simulink model "six_plus_six_AcmsteeringV09_main_2lflm"  (R2014a)
settings: Solver=FixedStepDiscrete  StartTime=0.0  StopTime=10.0  FixedStep=0.0005  RelTol=1e-3
InitFcn:
  | Veh_Par_wxt
undefined symbols (not defined in the file or in its folder): acc_spdctl, ag_thr, B, bra_em, bra_pre_gz2, bra_pre_gz34, bra_pre_yd, brakepre_dem_data, brakeTrq_dem_data, bratrq_max, ecucoder_acal, eff_tran, ESP_switch, G, guzhang_lf, guzhang_lm, guzhang_lr, guzhang_rf, guzhang_rm, guzhang_rr, kd1, kd2, ki1, ki2, kp1, kp2, L, myFIS, premax, Radius, RC_switch, s_opt_yi, s_opt_zhuan, s_opt_zhuan_add, s_opt_zhuan_table, spd_map_mot, spd_spdctl, speed_thr_park, TCS_switch, tras_ratio, trq_map_mot, trqmax_yd, trqmax_zx, trqmaxneg, v_gain, v_table, v_thr_park, zhidong_bianmazhi, zhidong_down, zhidong_up, zhidong_youmen, zhuanxiang_bianmazhi, zhuanxiang_down, zhuanxiang_up, zhuanxiang_youmen
libraries: simulink x980, ec5744lib x59, fuzblock x2
(part 15 of 25)

== matlab function six_plus_six_AcmsteeringV09_main_2lflm/MainControl/mode_control/backward/backward/Drive/驱动防滑控制TCS/直行TCS/直行/MATLAB Function ==
  data: s_act_lf input; flag_lf output; s_opt_zhuan input; s_opt_zhuan_add input; flag_lf_pre input int8
function flag_lf = fcn(s_act_lf,s_opt_zhuan,s_opt_zhuan_add,flag_lf_pre)
%#codegen
if s_act_lf>s_opt_zhuan+s_opt_zhuan_add
    flag_lf=int8(1);
elseif s_act_lf<s_opt_zhuan
    flag_lf =int8(0);
else
    flag_lf=int8(flag_lf_pre);
end
end

== matlab function six_plus_six_AcmsteeringV09_main_2lflm/MainControl/mode_control/backward/backward/Drive/驱动防滑控制TCS/直行TCS/直行/MATLAB Function6 ==
  data: s_act_rm input; flag_rm output; s_opt_zhuan input; s_opt_zhuan_add input; flag_rm_pre input int8
function flag_rm = fcn(s_act_rm,s_opt_zhuan,s_opt_zhuan_add,flag_rm_pre)
%#codegen
if s_act_rm>s_opt_zhuan+s_opt_zhuan_add
    flag_rm=int8(1);
elseif s_act_rm<s_opt_zhuan
    flag_rm =int8(0);
else
    flag_rm=int8(flag_rm_pre);
end
end

== matlab function six_plus_six_AcmsteeringV09_main_2lflm/Data_input/5/Enabled
Subsystem/MATLAB Function ==
  data: data1 input; y output; data2 input; data3 input; data4 input
function y = fcn(data1,data2,data3,data4)
%#codegen
y1=data4*256^3+data3*256^2+data2*256+data1;
y=typecast(uint32(y1),'single');
end
% y = u;

== matlab function six_plus_six_AcmsteeringV09_main_2lflm/Data_input/8/Enabled
Subsystem/MATLAB Function1 ==
  data: data1 input; y output; data2 input; data3 input; data4 input
function y = fcn(data1,data2,data3,data4)
%#codegen
y1=data4*256^3+data3*256^2+data2*256+data1;
y=typecast(uint32(y1),'single');
end
% y = u;

== matlab function six_plus_six_AcmsteeringV09_main_2lflm/MainControl/mode_control/backward/backward/Drive/MATLAB Function ==
  data: acc_y input; y output; ag_thr input
function y = fcn(acc_y,ag_thr)
%#codegen
if abs(acc_y)>=ag_thr
    y=int8(0);
else 
    y=int8(1);
end
end

== matlab function six_plus_six_AcmsteeringV09_main_2lflm/MainControl/mode_control/forward/forward/Drive/驱动防滑控制TCS/直行TCS/直行/MATLAB Function5 ==
  data: TCS_switch input; flag_lf1 output; flag_lm1 output; flag_lf input; flag_lm input; flag_lr input; flag_lr1 output; flag_rf input; flag_rm input; flag_rr input; flag_rf1 output; flag_rm1 output; flag_rr1 output
 function [flag_lf1,flag_lm1,flag_lr1,flag_rf1,flag_rm1,flag_rr1] = fcn(TCS_switch,flag_lf,flag_lm,flag_lr,flag_rf,flag_rm,flag_rr)
%#codegen
if TCS_switch==0
    flag_lf1=single(0);
    flag_lm1=single(0);
    flag_lr1=single(0);
    flag_rf1=single(0);
    flag_rm1=single(0);
    flag_rr1=single(0);
else
    flag_lf1=single(flag_lf);
    flag_lm1=single(flag_lm);
    flag_lr1=single(flag_lr);
    flag_rf1=single(flag_rf);
    flag_rm1=single(flag_rm);
    flag_rr1=single(flag_rr);
end
end

== system six_plus_six_AcmsteeringV09_main_2lflm/Data_input/RemoteControl1/Yaokong2 ==
  input : Inport
  Enable : EnablePort
  Demux : Demux  Outputs=8
  LIFEspan_Ad : Sum
  LIFEspan_Convert : DataTypeConversion  OutDataTypeStr=uint32
  LIFEspan_F : Gain
  LIFEspan_L : simulink/Logic and Bit Operations/Bitwise Operator  logicop=AND  UseBitMask=on  BitMask=255  BitMaskRealWorld=Stored Integer
  LIFEspan_O : Constant  Value=0  OutDataTypeStr=single
  LIFEspan_S : ArithShift
  LIFEspan_Sub : Subsystem
  LIFEspan_sat : Saturate  UpperLimit=255  LowerLimit=0
  LIFEspancv : DataTypeConversion
  SA_Ad : Sum
  SA_Convert : DataTypeConversion  OutDataTypeStr=uint32
  SA_F : Gain
  SA_L : simulink/Logic and Bit Operations/Bitwise Operator  logicop=AND  UseBitMask=on  BitMask=255  BitMaskRealWorld=Stored Integer
  SA_O : Constant  Value=0  OutDataTypeStr=single
  SA_S : ArithShift
  SA_Sub : Subsystem
  SA_sat : Saturate  UpperLimit=255  LowerLimit=0
  SAcv : DataTypeConversion
  SD_Ad : Sum
  SD_Convert : DataTypeConversion  OutDataTypeStr=uint32
  SD_F : Gain
  SD_L : simulink/Logic and Bit Operations/Bitwise Operator  logicop=AND  UseBitMask=on  BitMask=255  BitMaskRealWorld=Stored Integer
  SD_O : Constant  Value=0  OutDataTypeStr=single
  SD_S : ArithShift
  SD_Sub : Subsystem
  SD_sat : Saturate  UpperLimit=255  LowerLimit=0
  SDcv : DataTypeConversion
  SE_Ad : Sum
  SE_Convert : DataTypeConversion  OutDataTypeStr=uint32
  SE_F : Gain
  SE_L : simulink/Logic and Bit Operations/Bitwise Operator  logicop=AND  UseBitMask=on  BitMask=255  BitMaskRealWorld=Stored Integer
  SE_O : Constant  Value=0  OutDataTypeStr=single
  SE_S : ArithShift
  SE_Sub : Subsystem
  SE_sat : Saturate  UpperLimit=255  LowerLimit=0
  SEcv : DataTypeConversion
  SH_Ad : Sum
  SH_Convert : DataTypeConversion  OutDataTypeStr=uint32
  SH_F : Gain
  SH_L : simulink/Logic and Bit Operations/Bitwise Operator  logicop=AND  UseBitMask=on  BitMask=255  BitMaskRealWorld=Stored Integer
  SH_O : Constant  Value=0  OutDataTypeStr=single
  SH_S : ArithShift
  SH_Sub : Subsystem
  SH_sat : Saturate  UpperLimit=255  LowerLimit=0
  SHcv : DataTypeConversion
  SH_Out : Outport
  SE_Out : Outport  Port=2
  SD_Out : Outport  Port=3
  SA_Out : Outport  Port=4
  LIFEspan_Out : Outport  Port=5
  wires:
  SH_F/1 -> SH_Ad/1
  SH_O/1 -> SH_Ad/2
  SH_Ad/1 -> SH_sat/1
  SH_sat/1 -> SH_Out/1
  Demux/1 -> SH_Sub/1(In1)
  SH_Sub/1(Out1) -> SH_Convert/1
  SH_Convert/1 -> SH_L/1
  SH_L/1 -> SH_S/1
  SH_S/1 -> SHcv/1
  SHcv/1 -> SH_F/1
  SE_F/1 -> SE_Ad/1
  SE_O/1 -> SE_Ad/2
  SE_Ad/1 -> SE_sat/1
  SE_sat/1 -> SE_Out/1
  Demux/2 -> SE_Sub/1(In1)
  SE_Sub/1(Out1) -> SE_Convert/1
  SE_Convert/1 -> SE_L/1
  SE_L/1 -> SE_S/1
  SE_S/1 -> SEcv/1
  SEcv/1 -> SE_F/1
  SD_F/1 -> SD_Ad/1
  SD_O/1 -> SD_Ad/2
  SD_Ad/1 -> SD_sat/1
  SD_sat/1 -> SD_Out/1
  Demux/3 -> SD_Sub/1(In1)
  SD_Sub/1(Out1) -> SD_Convert/1
  SD_Convert/1 -> SD_L/1
  SD_L/1 -> SD_S/1
  SD_S/1 -> SDcv/1
  SDcv/1 -> SD_F/1
  SA_F/1 -> SA_Ad/1
  SA_O/1 -> SA_Ad/2
  SA_Ad/1 -> SA_sat/1
  SA_sat/1 -> SA_Out/1
  Demux/4 -> SA_Sub/1(In1)
  SA_Sub/1(Out1) -> SA_Convert/1
  SA_Convert/1 -> SA_L/1
  SA_L/1 -> SA_S/1
  SA_S/1 -> SAcv/1
  SAcv/1 -> SA_F/1
  LIFEspan_F/1 -> LIFEspan_Ad/1
  LIFEspan_O/1 -> LIFEspan_Ad/2
  LIFEspan_Ad/1 -> LIFEspan_sat/1
  LIFEspan_sat/1 -> LIFEspan_Out/1
  Demux/5 -> LIFEspan_Sub/1(In1)
  LIFEspan_Sub/1(Out1) -> LIFEspan_Convert/1
  LIFEspan_Convert/1 -> LIFEspan_L/1
  LIFEspan_L/1 -> LIFEspan_S/1
  LIFEspan_S/1 -> LIFEspancv/1
  LIFEspancv/1 -> LIFEspan_F/1
  input/1 -> Demux/1

== system six_plus_six_AcmsteeringV09_main_2lflm/Data_input/RemoteControl2/Yaokong1 ==
  input : Inport
  Enable : EnablePort
  Data Type Conversion : DataTypeConversion
  Data Type Conversion1 : DataTypeConversion
  Demux : Demux  Outputs=8
  Leftstick_leftright_Ad : Sum
  Leftstick_leftright_Convert : DataTypeConversion  OutDataTypeStr=uint32
  Leftstick_leftright_F : Gain
  Leftstick_leftright_L : simulink/Logic and Bit Operations/Bitwise Operator  logicop=AND  UseBitMask=on  BitMask=65535  BitMaskRealWorld=Stored Integer
  Leftstick_leftright_O : Constant  Value=0  OutDataTypeStr=single
  Leftstick_leftright_S : ArithShift
  Leftstick_leftright_Sub : Subsystem
  Leftstick_leftright_sat : Saturate  UpperLimit=65535  LowerLimit=0
  Leftstick_leftrightcv : DataTypeConversion
  Leftstick_leftrightinput1_Ad : Sum
  Leftstick_leftrightinput1_C : Constant  Value=256
  Leftstick_leftrightinput1_P : Product
  Leftstick_updown_Ad : Sum
  Leftstick_updown_Convert : DataTypeConversion  OutDataTypeStr=uint32
  Leftstick_updown_F : Gain
  Leftstick_updown_L : simulink/Logic and Bit Operations/Bitwise Operator  logicop=AND  UseBitMask=on  BitMask=65535  BitMaskRealWorld=Stored Integer
  Leftstick_updown_O : Constant  Value=0  OutDataTypeStr=single
  Leftstick_updown_S : ArithShift
  Leftstick_updown_Sub : Subsystem
  Leftstick_updown_sat : Saturate  UpperLimit=65535  LowerLimit=0
  Leftstick_updowncv : DataTypeConversion
  Leftstick_updowninput3_Ad : Sum
  Leftstick_updowninput3_C : Constant  Value=256
  Leftstick_updowninput3_P : Product
  Rightstick_leftright_Ad : Sum
  Rightstick_leftright_Convert : DataTypeConversion  OutDataTypeStr=uint32
  Rightstick_leftright_F : Gain
  Rightstick_leftright_L : simulink/Logic and Bit Operations/Bitwise Operator  logicop=AND  UseBitMask=on  BitMask=65535  BitMaskRealWorld=Stored Integer
  Rightstick_leftright_O : Constant  Value=0  OutDataTypeStr=single
  Rightstick_leftright_S : ArithShift
  Rightstick_leftright_Sub : Subsystem
  Rightstick_leftright_sat : Saturate  UpperLimit=65535  LowerLimit=0
  Rightstick_leftrightcv : DataTypeConversion
  Rightstick_leftrightinput5_Ad : Sum
  Rightstick_leftrightinput5_C : Constant  Value=256
  Rightstick_leftrightinput5_P : Product
  Rightstick_updown_Ad : Sum
  Rightstick_updown_Convert : DataTypeConversion  OutDataTypeStr=uint32
  Rightstick_updown_F : Gain
  Rightstick_updown_L : simulink/Logic and Bit Operations/Bitwise Operator  logicop=AND  UseBitMask=on  BitMask=65535  BitMaskRealWorld=Stored Integer
  Rightstick_updown_O : Constant  Value=0  OutDataTypeStr=single
  Rightstick_updown_S : ArithShift
  Rightstick_updown_Sub : Subsystem
  Rightstick_updown_sat : Saturate  UpperLimit=65535  LowerLimit=0
  Rightstick_updowncv : DataTypeConversion
  Rightstick_updowninput7_Ad : Sum
  Rightstick_updowninput7_C : Constant  Value=256
  Rightstick_updowninput7_P : Product
  Rightstick_updown_Out : Outport
  Rightstick_leftright_Out : Outport  Port=2
  Leftstick_updown_Out : Outport  Port=3
  Leftstick_leftright_Out : Outport  Port=4
  wires:
  Rightstick_updown_F/1 -> Rightstick_updown_Ad/1
  Rightstick_updown_O/1 -> Rightstick_updown_Ad/2
  Rightstick_updown_Ad/1 -> Rightstick_updown_sat/1
  Rightstick_updown_sat/1 -> Rightstick_updown_Out/1
  Demux/7 -> Rightstick_updowninput7_P/1
  Rightstick_updowninput7_C/1 -> Rightstick_updowninput7_P/2
  Rightstick_updowninput7_P/1 -> Rightstick_updowninput7_Ad/1
  Demux/8 -> Rightstick_updowninput7_Ad/2
  Rightstick_updowninput7_Ad/1 -> Rightstick_updown_Sub/1(In1)
  Rightstick_updown_Sub/1(Out1) -> Rightstick_updown_Convert/1
  Rightstick_updown_Convert/1 -> Rightstick_updown_L/1
  Rightstick_updown_L/1 -> Rightstick_updown_S/1
  Rightstick_updown_S/1 -> Rightstick_updowncv/1
  Rightstick_updowncv/1 -> Rightstick_updown_F/1
  Rightstick_leftright_F/1 -> Rightstick_leftright_Ad/1
  Rightstick_leftright_O/1 -> Rightstick_leftright_Ad/2
  Rightstick_leftright_Ad/1 -> Rightstick_leftright_sat/1
  Rightstick_leftright_sat/1 -> Rightstick_leftright_Out/1
  Demux/5 -> Rightstick_leftrightinput5_P/1
  Rightstick_leftrightinput5_C/1 -> Rightstick_leftrightinput5_P/2
  Rightstick_leftrightinput5_P/1 -> Rightstick_leftrightinput5_Ad/1
  Demux/6 -> Rightstick_leftrightinput5_Ad/2
  Rightstick_leftrightinput5_Ad/1 -> Rightstick_leftright_Sub/1(In1)
  Rightstick_leftright_Sub/1(Out1) -> Rightstick_leftright_Convert/1
  Rightstick_leftright_Convert/1 -> Rightstick_leftright_L/1
  Rightstick_leftright_L/1 -> Rightstick_leftright_S/1
  Rightstick_leftright_S/1 -> Rightstick_leftrightcv/1
  Rightstick_leftrightcv/1 -> Rightstick_leftright_F/1
  Leftstick_updown_F/1 -> Leftstick_updown_Ad/1
  Leftstick_updown_O/1 -> Leftstick_updown_Ad/2
  Leftstick_updown_Ad/1 -> Leftstick_updown_sat/1
  Leftstick_updown_sat/1 -> Leftstick_updown_Out/1
  Demux/3 -> Data Type Conversion/1
  Leftstick_updowninput3_C/1 -> Leftstick_updowninput3_P/2
  Leftstick_updowninput3_P/1 -> Leftstick_updowninput3_Ad/1
  Demux/4 -> Data Type Conversion1/1
  Leftstick_updowninput3_Ad/1 -> Leftstick_updown_Sub/1(In1)
  Leftstick_updown_Sub/1(Out1) -> Leftstick_updown_Convert/1
  Leftstick_updown_Convert/1 -> Leftstick_updown_L/1
  Leftstick_updown_L/1 -> Leftstick_updown_S/1
  Leftstick_updown_S/1 -> Leftstick_updowncv/1
  Leftstick_updowncv/1 -> Leftstick_updown_F/1
  Leftstick_leftright_F/1 -> Leftstick_leftright_Ad/1
  Leftstick_leftright_O/1 -> Leftstick_leftright_Ad/2
  Leftstick_leftright_Ad/1 -> Leftstick_leftright_sat/1
  Leftstick_leftright_sat/1 -> Leftstick_leftright_Out/1
  Demux/1 -> Leftstick_leftrightinput1_P/1
  Leftstick_leftrightinput1_C/1 -> Leftstick_leftrightinput1_P/2
  Leftstick_leftrightinput1_P/1 -> Leftstick_leftrightinput1_Ad/1
  Demux/2 -> Leftstick_leftrightinput1_Ad/2
  Leftstick_leftrightinput1_Ad/1 -> Leftstick_leftright_Sub/1(In1)
  Leftstick_leftright_Sub/1(Out1) -> Leftstick_leftright_Convert/1
  Leftstick_leftright_Convert/1 -> Leftstick_leftright_L/1
  Leftstick_leftright_L/1 -> Leftstick_leftright_S/1
  Leftstick_leftright_S/1 -> Leftstick_leftrightcv/1
  Leftstick_leftrightcv/1 -> Leftstick_leftright_F/1
  input/1 -> Demux/1
  Data Type Conversion/1 -> Leftstick_updowninput3_P/1
  Data Type Conversion1/1 -> Leftstick_updowninput3_Ad/2

== system six_plus_six_AcmsteeringV09_main_2lflm/MainControl/mode_control/Park ==
  Signals : Inport
  Action Port : ActionPort  ActionType=case
  Mux : Mux  Inputs=10
  park : Subsystem
  park_dem : Outport
  wires:
  Signals/1 -> park/1(Signals)
  Mux/1 -> park_dem/1
  park/9(motec_position_3) -> Mux/9
  park/10(motec_position_4) -> Mux/10
  park/1(mot_lf) -> Mux/1
  park/2(mot_lm) -> Mux/2
  park/5(mot_rm) -> Mux/5
  park/4(mot_rf) -> Mux/4
  park/3(mot_lr) -> Mux/3
  park/7(motec_position_1) -> Mux/7
  park/8(motec_position_2) -> Mux/8
  park/6(mot_rr) -> Mux/6

== system six_plus_six_AcmsteeringV09_main_2lflm/MainControl/mode_control/backward ==
  Signals : Inport
  Action Port : ActionPort  ActionType=case
  backward : Subsystem
  backward_dem : Outport
  wires:
  Signals/1 -> backward/1(Signals)
  backward/1(backward_dem) -> backward_dem/1

== system six_plus_six_AcmsteeringV09_main_2lflm/MainControl/mode_control/center_steer ==
  Signals : Inport
  Action Port : ActionPort  ActionType=case
  Mux : Mux  Inputs=10
  center_steer : Subsystem
  center_steer_dem : Outport
  wires:
  Mux/1 -> center_steer_dem/1
  Signals/1 -> center_steer/1(Signals)
  center_steer/6(mot_rr) -> Mux/6
  center_steer/1(mot_lf) -> Mux/1
  center_steer/4(mot_rf) -> Mux/4
  center_steer/3(mot_lr) -> Mux/3
  center_steer/5(mot_rm) -> Mux/5
  center_steer/2(mot_lm) -> Mux/2
  center_steer/7(motec_position_1) -> Mux/7
  center_steer/8(motec_position_2) -> Mux/8
  center_steer/10(motec_position_4) -> Mux/10
  center_steer/9(motec_position_3) -> Mux/9

== system six_plus_six_AcmsteeringV09_main_2lflm/MainControl/mode_control/emergency_stop ==
  Signals : Inport
  Action Port : ActionPort  ActionType=case
  Mux : Mux  Inputs=10
  emergency_stop : Subsystem
  emergency_stop_dem : Outport
  wires:
  Mux/1 -> emergency_stop_dem/1
  Signals/1 -> emergency_stop/1(Signals)
  emergency_stop/8(motec_position_2) -> Mux/8
  emergency_stop/9(motec_position_3) -> Mux/9
  emergency_stop/10(motec_position_4) -> Mux/10
  emergency_stop/7(motec_position_1) -> Mux/7
  emergency_stop/3(mot_lr) -> Mux/3
  emergency_stop/1(mot_lf) -> Mux/1
  emergency_stop/2(mot_lm) -> Mux/2
  emergency_stop/5(mot_rm) -> Mux/5
  emergency_stop/6(mot_rr) -> Mux/6
  emergency_stop/4(mot_rf) -> Mux/4

== system six_plus_six_AcmsteeringV09_main_2lflm/MainControl/mode_control/forward ==
  Signals : Inport
  Action Port : ActionPort  ActionType=case
  forward : Subsystem
  forward_dem : Outport
  wires:
  Signals/1 -> forward/1(Signals)
  forward/1(forward_dem) -> forward_dem/1

== system six_plus_six_AcmsteeringV09_main_2lflm/MainControl/mode_control/neutral ==
  Signals : Inport
  Action Port : ActionPort  ActionType=case
  Mux : Mux  Inputs=10
  neutral : Subsystem
  neutral_dem : Outport
  wires:
  Mux/1 -> neutral_dem/1
  Signals/1 -> neutral/1(Signals)
  neutral/3(mot_lr) -> Mux/3
  neutral/5(mot_rm) -> Mux/5
  neutral/6(mot_rr) -> Mux/6
  neutral/2(mot_lm) -> Mux/2
  neutral/1(mot_lf) -> Mux/1
  neutral/4(mot_rf) -> Mux/4
  neutral/7(motec_position_1) -> Mux/7
  neutral/8(motec_position_2) -> Mux/8
  neutral/10(motec_position_4) -> Mux/10
  neutral/9(motec_position_3) -> Mux/9

== system six_plus_six_AcmsteeringV09_main_2lflm/Subsystem/VCU1/VCU1_CtrlModel ==
  VCU1_CtrlModel : Inport
  Constant{2..8} (7 alike) : Constant  Value=0  OutDataTypeStr=uint8
  VCU1_CtrlModelRon : Rounding  Operator=round
  VCU1_CtrlModel_1sat : Saturate  UpperLimit=4  LowerLimit=0
  VCU1_CtrlModel_Convert : DataTypeConversion  OutDataTypeStr=uint8
  VCU1_CtrlModel_Convert1 : DataTypeConversion  OutDataTypeStr=uint32
  VCU1_CtrlModel_D : Product  Inputs=*/
  VCU1_CtrlModel_F : Constant  OutDataTypeStr=single
  VCU1_CtrlModel_L : simulink/Logic and Bit Operations/Bitwise Operator  logicop=AND  UseBitMask=on  BitMask=4  BitMaskRealWorld=Stored Integer
  VCU1_CtrlModel_O : Constant  Value=0  OutDataTypeStr=single
  VCU1_CtrlModel_S : ArithShift  BitShiftNumber=-2
  VCU1_CtrlModel_sat : Saturate  UpperLimit=1  LowerLimit=0
  VCU1_CtrlModel_st : Sum  Inputs=+-
  output1 : Outport
  output2 : Outport  Port=2
  output3 : Outport  Port=3
  output4 : Outport  Port=4
  output5 : Outport  Port=5
  output6 : Outport  Port=6
  output7 : Outport  Port=7
  output8 : Outport  Port=8
  wires:
  VCU1_CtrlModel/1 -> VCU1_CtrlModel_sat/1
  VCU1_CtrlModel_sat/1 -> VCU1_CtrlModel_st/1
  VCU1_CtrlModel_O/1 -> VCU1_CtrlModel_st/2
  VCU1_CtrlModel_st/1 -> VCU1_CtrlModel_D/1
  VCU1_CtrlModel_F/1 -> VCU1_CtrlModel_D/2
  VCU1_CtrlModel_D/1 -> VCU1_CtrlModelRon/1
  VCU1_CtrlModelRon/1 -> VCU1_CtrlModel_S/1
  VCU1_CtrlModel_S/1 -> VCU1_CtrlModel_1sat/1
  VCU1_CtrlModel_1sat/1 -> VCU1_CtrlModel_Convert1/1
  VCU1_CtrlModel_Convert1/1 -> VCU1_CtrlModel_L/1
  VCU1_CtrlModel_L/1 -> VCU1_CtrlModel_Convert/1
  VCU1_CtrlModel_Convert/1 -> output1/1
  Constant2/1 -> output2/1
  Constant3/1 -> output3/1
  Constant4/1 -> output4/1
  Constant5/1 -> output5/1
  Constant6/1 -> output6/1
  Constant7/1 -> output7/1
  Constant8/1 -> output8/1

== system six_plus_six_AcmsteeringV09_main_2lflm/Subsystem/VCU1/VCU1_EnableReq ==
  VCU1_EnableReq : Inport
  Constant{2..8} (7 alike) : Constant  Value=0  OutDataTypeStr=uint8
  VCU1_EnableReqRon : Rounding  Operator=round
  VCU1_EnableReq_1sat : Saturate  UpperLimit=3  LowerLimit=0
  VCU1_EnableReq_Convert : DataTypeConversion  OutDataTypeStr=uint8
  VCU1_EnableReq_Convert1 : DataTypeConversion  OutDataTypeStr=uint32
  VCU1_EnableReq_D : Product  Inputs=*/
  VCU1_EnableReq_F : Constant  OutDataTypeStr=single
  VCU1_EnableReq_L : simulink/Logic and Bit Operations/Bitwise Operator  logicop=AND  UseBitMask=on  BitMask=3  BitMaskRealWorld=Stored Integer
  VCU1_EnableReq_O : Constant  Value=0  OutDataTypeStr=single
  VCU1_EnableReq_S : ArithShift
  VCU1_EnableReq_sat : Saturate  UpperLimit=3  LowerLimit=0
  VCU1_EnableReq_st : Sum  Inputs=+-
  output1 : Outport
  output2 : Outport  Port=2
  output3 : Outport  Port=3
  output4 : Outport  Port=4
  output5 : Outport  Port=5
  output6 : Outport  Port=6
  output7 : Outport  Port=7
  output8 : Outport  Port=8
  wires:
  VCU1_EnableReq/1 -> VCU1_EnableReq_sat/1
  VCU1_EnableReq_sat/1 -> VCU1_EnableReq_st/1
  VCU1_EnableReq_O/1 -> VCU1_EnableReq_st/2
  VCU1_EnableReq_st/1 -> VCU1_EnableReq_D/1
  VCU1_EnableReq_F/1 -> VCU1_EnableReq_D/2
  VCU1_EnableReq_D/1 -> VCU1_EnableReqRon/1
  VCU1_EnableReqRon/1 -> VCU1_EnableReq_S/1
  VCU1_EnableReq_S/1 -> VCU1_EnableReq_1sat/1
  VCU1_EnableReq_1sat/1 -> VCU1_EnableReq_Convert1/1
  VCU1_EnableReq_Convert1/1 -> VCU1_EnableReq_L/1
  VCU1_EnableReq_L/1 -> VCU1_EnableReq_Convert/1
  VCU1_EnableReq_Convert/1 -> output1/1
  Constant2/1 -> output2/1
  Constant3/1 -> output3/1
  Constant4/1 -> output4/1
  Constant5/1 -> output5/1
  Constant6/1 -> output6/1
  Constant7/1 -> output7/1
  Constant8/1 -> output8/1

== system six_plus_six_AcmsteeringV09_main_2lflm/Subsystem/VCU1/VCU1_GearCmd ==
  VCU1_GearCmd : Inport
  Constant{2..8} (7 alike) : Constant  Value=0  OutDataTypeStr=uint8
  VCU1_GearCmdRon : Rounding  Operator=round
  VCU1_GearCmd_1sat : Saturate  UpperLimit=24  LowerLimit=0
  VCU1_GearCmd_Convert : DataTypeConversion  OutDataTypeStr=uint8
  VCU1_GearCmd_Convert1 : DataTypeConversion  OutDataTypeStr=uint32
  VCU1_GearCmd_D : Product  Inputs=*/
  VCU1_GearCmd_F : Constant  OutDataTypeStr=single
  VCU1_GearCmd_L : simulink/Logic and Bit Operations/Bitwise Operator  logicop=AND  UseBitMask=on  BitMask=24  BitMaskRealWorld=Stored Integer
  VCU1_GearCmd_O : Constant  Value=0  OutDataTypeStr=single
  VCU1_GearCmd_S : ArithShift  BitShiftNumber=-3
  VCU1_GearCmd_sat : Saturate  UpperLimit=3  LowerLimit=0
  VCU1_GearCmd_st : Sum  Inputs=+-
  output1 : Outport
  output2 : Outport  Port=2
  output3 : Outport  Port=3
  output4 : Outport  Port=4
  output5 : Outport  Port=5
  output6 : Outport  Port=6
  output7 : Outport  Port=7
  output8 : Outport  Port=8
  wires:
  VCU1_GearCmd/1 -> VCU1_GearCmd_sat/1
  VCU1_GearCmd_sat/1 -> VCU1_GearCmd_st/1
  VCU1_GearCmd_O/1 -> VCU1_GearCmd_st/2
  VCU1_GearCmd_st/1 -> VCU1_GearCmd_D/1
  VCU1_GearCmd_F/1 -> VCU1_GearCmd_D/2
  VCU1_GearCmd_D/1 -> VCU1_GearCmdRon/1
  VCU1_GearCmdRon/1 -> VCU1_GearCmd_S/1
  VCU1_GearCmd_S/1 -> VCU1_GearCmd_1sat/1
  VCU1_GearCmd_1sat/1 -> VCU1_GearCmd_Convert1/1
  VCU1_GearCmd_Convert1/1 -> VCU1_GearCmd_L/1
  VCU1_GearCmd_L/1 -> VCU1_GearCmd_Convert/1
  VCU1_GearCmd_Convert/1 -> output1/1
  Constant2/1 -> output2/1
  Constant3/1 -> output3/1
  Constant4/1 -> output4/1
  Constant5/1 -> output5/1
  Constant6/1 -> output6/1
  Constant7/1 -> output7/1
  Constant8/1 -> output8/1

== system six_plus_six_AcmsteeringV09_main_2lflm/Subsystem/VCU1/VCU1_LifeCnt ==
  VCU1_LifeCnt : Inport
  Constant{1..7} (7 alike) : Constant  Value=0  OutDataTypeStr=uint8
  VCU1_LifeCntRon : Rounding  Operator=round
  VCU1_LifeCnt_1sat : Saturate  UpperLimit=255  LowerLimit=0
  VCU1_LifeCnt_Convert : DataTypeConversion  OutDataTypeStr=uint8
  VCU1_LifeCnt_Convert1 : DataTypeConversion  OutDataTypeStr=uint32
  VCU1_LifeCnt_D : Product  Inputs=*/
  VCU1_LifeCnt_F : Constant  OutDataTypeStr=single
  VCU1_LifeCnt_L : simulink/Logic and Bit Operations/Bitwise Operator  logicop=AND  UseBitMask=on  BitMask=255  BitMaskRealWorld=Stored Integer
  VCU1_LifeCnt_O : Constant  Value=0  OutDataTypeStr=single
  VCU1_LifeCnt_S : ArithShift
  VCU1_LifeCnt_sat : Saturate  UpperLimit=255  LowerLimit=0
  VCU1_LifeCnt_st : Sum  Inputs=+-
  output1 : Outport
  output2 : Outport  Port=2
  output3 : Outport  Port=3
  output4 : Outport  Port=4
  output5 : Outport  Port=5
  output6 : Outport  Port=6
  output7 : Outport  Port=7
  output8 : Outport  Port=8
  wires:
  VCU1_LifeCnt/1 -> VCU1_LifeCnt_sat/1
  VCU1_LifeCnt_sat/1 -> VCU1_LifeCnt_st/1
  VCU1_LifeCnt_O/1 -> VCU1_LifeCnt_st/2
  VCU1_LifeCnt_st/1 -> VCU1_LifeCnt_D/1
  VCU1_LifeCnt_F/1 -> VCU1_LifeCnt_D/2
  VCU1_LifeCnt_D/1 -> VCU1_LifeCntRon/1
  VCU1_LifeCntRon/1 -> VCU1_LifeCnt_S/1
  VCU1_LifeCnt_S/1 -> VCU1_LifeCnt_1sat/1
  VCU1_LifeCnt_1sat/1 -> VCU1_LifeCnt_Convert1/1
  VCU1_LifeCnt_Convert1/1 -> VCU1_LifeCnt_L/1
  VCU1_LifeCnt_L/1 -> VCU1_LifeCnt_Convert/1
  VCU1_LifeCnt_Convert/1 -> output8/1
  Constant1/1 -> output1/1
  Constant2/1 -> output2/1
  Constant3/1 -> output3/1
  Constant4/1 -> output4/1
  Constant5/1 -> output5/1
  Constant6/1 -> output6/1
  Constant7/1 -> output7/1

== system six_plus_six_AcmsteeringV09_main_2lflm/Subsystem/VCU1/VCU1_SpeedMax ==
  VCU1_SpeedMax : Inport
  Constant{1,4..8} (6 alike) : Constant  Value=0  OutDataTypeStr=uint8
  VCU1_SpeedMaxBitCov : DataTypeConversion  OutDataTypeStr=uint8
  VCU1_SpeedMaxCOV : DataTypeConversion  OutDataTypeStr=uint8
  VCU1_SpeedMaxRon : Rounding  Operator=round
  VCU1_SpeedMax_1sat : Saturate  UpperLimit=65535  LowerLimit=0
  VCU1_SpeedMax_And : simulink/Logic and Bit Operations/Bitwise Operator  logicop=AND  UseBitMask=off  NumInputPorts=2  BitMask=bin2dec('11011001')  BitMaskRealWorld=Stored Integer
  VCU1_SpeedMax_And_C : Constant  Value=255  OutDataTypeStr=uint32
  VCU1_SpeedMax_Convert : DataTypeConversion  OutDataTypeStr=uint32
  VCU1_SpeedMax_D : Product  Inputs=*/
  VCU1_SpeedMax_D1 : Product  Inputs=*/
  VCU1_SpeedMax_F : Constant  OutDataTypeStr=single
  VCU1_SpeedMax_L : simulink/Logic and Bit Operations/Bitwise Operator  logicop=AND  UseBitMask=on  BitMask=65535  BitMaskRealWorld=Stored Integer
  VCU1_SpeedMax_O : Constant  Value=0  OutDataTypeStr=single
  VCU1_SpeedMax_S : ArithShift
  VCU1_SpeedMax_sat : Saturate  UpperLimit=10000  LowerLimit=0
  VCU1_SpeedMax_st : Sum  Inputs=+-
  VCU1_SpeedMaxoutput2_C : Constant  Value=256
  output1 : Outport
  output2 : Outport  Port=2
  output3 : Outport  Port=3
  output4 : Outport  Port=4
  output5 : Outport  Port=5
  output6 : Outport  Port=6
  output7 : Outport  Port=7
  output8 : Outport  Port=8
  wires:
  VCU1_SpeedMax/1 -> VCU1_SpeedMax_sat/1
  VCU1_SpeedMax_sat/1 -> VCU1_SpeedMax_st/1
  VCU1_SpeedMax_O/1 -> VCU1_SpeedMax_st/2
  VCU1_SpeedMax_st/1 -> VCU1_SpeedMax_D/1
  VCU1_SpeedMax_F/1 -> VCU1_SpeedMax_D/2
  VCU1_SpeedMax_D/1 -> VCU1_SpeedMaxRon/1
  VCU1_SpeedMaxRon/1 -> VCU1_SpeedMax_S/1
  VCU1_SpeedMax_S/1 -> VCU1_SpeedMax_1sat/1
  VCU1_SpeedMax_1sat/1 -> VCU1_SpeedMax_Convert/1
  VCU1_SpeedMax_Convert/1 -> VCU1_SpeedMax_L/1
  VCU1_SpeedMax_L/1 -> VCU1_SpeedMax_D1/1, VCU1_SpeedMax_And/1
  VCU1_SpeedMaxoutput2_C/1 -> VCU1_SpeedMax_D1/2
  VCU1_SpeedMax_D1/1 -> VCU1_SpeedMaxCOV/1
  VCU1_SpeedMaxCOV/1 -> output2/1
  VCU1_SpeedMax_And_C/1 -> VCU1_SpeedMax_And/2
  VCU1_SpeedMax_And/1 -> VCU1_SpeedMaxBitCov/1
  VCU1_SpeedMaxBitCov/1 -> output3/1
  Constant1/1 -> output1/1
  Constant4/1 -> output4/1
  Constant5/1 -> output5/1
  Constant6/1 -> output6/1
  Constant7/1 -> output7/1
  Constant8/1 -> output8/1

== system six_plus_six_AcmsteeringV09_main_2lflm/Subsystem/VCU1/VCU1_TorqueRef ==
  VCU1_TorqueRef : Inport
  Constant{1..3,6..8} (6 alike) : Constant  Value=0  OutDataTypeStr=uint8
  VCU1_TorqueRefBitCov : DataTypeConversion  OutDataTypeStr=uint8
  VCU1_TorqueRefCOV : DataTypeConversion  OutDataTypeStr=uint8
  VCU1_TorqueRefRon : Rounding  Operator=round
  VCU1_TorqueRef_1sat : Saturate  UpperLimit=65535  LowerLimit=0
  VCU1_TorqueRef_And : simulink/Logic and Bit Operations/Bitwise Operator  logicop=AND  UseBitMask=off  NumInputPorts=2  BitMask=bin2dec('11011001')  BitMaskRealWorld=Stored Integer
  VCU1_TorqueRef_And_C : Constant  Value=255  OutDataTypeStr=uint32
  VCU1_TorqueRef_Convert : DataTypeConversion  OutDataTypeStr=uint32
  VCU1_TorqueRef_D : Product  Inputs=*/
  VCU1_TorqueRef_D1 : Product  Inputs=*/
  VCU1_TorqueRef_F : Constant  Value=0.1  OutDataTypeStr=single
  VCU1_TorqueRef_L : simulink/Logic and Bit Operations/Bitwise Operator  logicop=AND  UseBitMask=on  BitMask=65535  BitMaskRealWorld=Stored Integer
  VCU1_TorqueRef_O : Constant  Value=-1000  OutDataTypeStr=single
  VCU1_TorqueRef_S : ArithShift
  VCU1_TorqueRef_sat : Saturate  UpperLimit=1000  LowerLimit=-1000
  VCU1_TorqueRef_st : Sum  Inputs=+-
  VCU1_TorqueRefoutput4_C : Constant  Value=256
  output1 : Outport
  output2 : Outport  Port=2
  output3 : Outport  Port=3
  output4 : Outport  Port=4
  output5 : Outport  Port=5
  output6 : Outport  Port=6
  output7 : Outport  Port=7
  output8 : Outport  Port=8
  wires:
  VCU1_TorqueRef/1 -> VCU1_TorqueRef_sat/1
  VCU1_TorqueRef_sat/1 -> VCU1_TorqueRef_st/1
  VCU1_TorqueRef_O/1 -> VCU1_TorqueRef_st/2
  VCU1_TorqueRef_st/1 -> VCU1_TorqueRef_D/1
  VCU1_TorqueRef_F/1 -> VCU1_TorqueRef_D/2
  VCU1_TorqueRef_D/1 -> VCU1_TorqueRefRon/1
  VCU1_TorqueRefRon/1 -> VCU1_TorqueRef_S/1
  VCU1_TorqueRef_S/1 -> VCU1_TorqueRef_1sat/1
  VCU1_TorqueRef_1sat/1 -> VCU1_TorqueRef_Convert/1
  VCU1_TorqueRef_Convert/1 -> VCU1_TorqueRef_L/1
  VCU1_TorqueRef_L/1 -> VCU1_TorqueRef_D1/1, VCU1_TorqueRef_And/1
  VCU1_TorqueRefoutput4_C/1 -> VCU1_TorqueRef_D1/2
  VCU1_TorqueRef_D1/1 -> VCU1_TorqueRefCOV/1
  VCU1_TorqueRefCOV/1 -> output4/1
  VCU1_TorqueRef_And_C/1 -> VCU1_TorqueRef_And/2
  VCU1_TorqueRef_And/1 -> VCU1_TorqueRefBitCov/1
  VCU1_TorqueRefBitCov/1 -> output5/1
  Constant1/1 -> output1/1
  Constant2/1 -> output2/1
  Constant3/1 -> output3/1
  Constant6/1 -> output6/1
  Constant7/1 -> output7/1
  Constant8/1 -> output8/1

== system six_plus_six_AcmsteeringV09_main_2lflm/Subsystem/VCU2/VCU1_CtrlModel ==
  VCU1_CtrlModel : Inport
  Constant{2..8} (7 alike) : Constant  Value=0  OutDataTypeStr=uint8
  VCU1_CtrlModelRon : Rounding  Operator=round
  VCU1_CtrlModel_1sat : Saturate  UpperLimit=4  LowerLimit=0
  VCU1_CtrlModel_Convert : DataTypeConversion  OutDataTypeStr=uint8
  VCU1_CtrlModel_Convert1 : DataTypeConversion  OutDataTypeStr=uint32
  VCU1_CtrlModel_D : Product  Inputs=*/
  VCU1_CtrlModel_F : Constant  OutDataTypeStr=single
  VCU1_CtrlModel_L : simulink/Logic and Bit Operations/Bitwise Operator  logicop=AND  UseBitMask=on  BitMask=4  BitMaskRealWorld=Stored Integer
  VCU1_CtrlModel_O : Constant  Value=0  OutDataTypeStr=single
  VCU1_CtrlModel_S : ArithShift  BitShiftNumber=-2
  VCU1_CtrlModel_sat : Saturate  UpperLimit=1  LowerLimit=0
  VCU1_CtrlModel_st : Sum  Inputs=+-
  output1 : Outport
  output2 : Outport  Port=2
  output3 : Outport  Port=3
  output4 : Outport  Port=4
  output5 : Outport  Port=5
  output6 : Outport  Port=6
  output7 : Outport  Port=7
  output8 : Outport  Port=8
  wires:
  VCU1_CtrlModel/1 -> VCU1_CtrlModel_sat/1
  VCU1_CtrlModel_sat/1 -> VCU1_CtrlModel_st/1
  VCU1_CtrlModel_O/1 -> VCU1_CtrlModel_st/2
  VCU1_CtrlModel_st/1 -> VCU1_CtrlModel_D/1
  VCU1_CtrlModel_F/1 -> VCU1_CtrlModel_D/2
  VCU1_CtrlModel_D/1 -> VCU1_CtrlModelRon/1
  VCU1_CtrlModelRon/1 -> VCU1_CtrlModel_S/1
  VCU1_CtrlModel_S/1 -> VCU1_CtrlModel_1sat/1
  VCU1_CtrlModel_1sat/1 -> VCU1_CtrlModel_Convert1/1
  VCU1_CtrlModel_Convert1/1 -> VCU1_CtrlModel_L/1
  VCU1_CtrlModel_L/1 -> VCU1_CtrlModel_Convert/1
  VCU1_CtrlModel_Convert/1 -> output1/1
  Constant2/1 -> output2/1
  Constant3/1 -> output3/1
  Constant4/1 -> output4/1
  Constant5/1 -> output5/1
  Constant6/1 -> output6/1
  Constant7/1 -> output7/1
  Constant8/1 -> output8/1

== system six_plus_six_AcmsteeringV09_main_2lflm/Subsystem/VCU2/VCU1_EnableReq ==
  VCU1_EnableReq : Inport
  Constant{2..8} (7 alike) : Constant  Value=0  OutDataTypeStr=uint8
  VCU1_EnableReqRon : Rounding  Operator=round
  VCU1_EnableReq_1sat : Saturate  UpperLimit=3  LowerLimit=0
  VCU1_EnableReq_Convert : DataTypeConversion  OutDataTypeStr=uint8
  VCU1_EnableReq_Convert1 : DataTypeConversion  OutDataTypeStr=uint32
  VCU1_EnableReq_D : Product  Inputs=*/
  VCU1_EnableReq_F : Constant  OutDataTypeStr=single
  VCU1_EnableReq_L : simulink/Logic and Bit Operations/Bitwise Operator  logicop=AND  UseBitMask=on  BitMask=3  BitMaskRealWorld=Stored Integer
  VCU1_EnableReq_O : Constant  Value=0  OutDataTypeStr=single
  VCU1_EnableReq_S : ArithShift
  VCU1_EnableReq_sat : Saturate  UpperLimit=3  LowerLimit=0
  VCU1_EnableReq_st : Sum  Inputs=+-
  output1 : Outport
  output2 : Outport  Port=2
  output3 : Outport  Port=3
  output4 : Outport  Port=4
  output5 : Outport  Port=5
  output6 : Outport  Port=6
  output7 : Outport  Port=7
  output8 : Outport  Port=8
  wires:
  VCU1_EnableReq/1 -> VCU1_EnableReq_sat/1
  VCU1_EnableReq_sat/1 -> VCU1_EnableReq_st/1
  VCU1_EnableReq_O/1 -> VCU1_EnableReq_st/2
  VCU1_EnableReq_st/1 -> VCU1_EnableReq_D/1
  VCU1_EnableReq_F/1 -> VCU1_EnableReq_D/2
  VCU1_EnableReq_D/1 -> VCU1_EnableReqRon/1
  VCU1_EnableReqRon/1 -> VCU1_EnableReq_S/1
  VCU1_EnableReq_S/1 -> VCU1_EnableReq_1sat/1
  VCU1_EnableReq_1sat/1 -> VCU1_EnableReq_Convert1/1
  VCU1_EnableReq_Convert1/1 -> VCU1_EnableReq_L/1
  VCU1_EnableReq_L/1 -> VCU1_EnableReq_Convert/1
  VCU1_EnableReq_Convert/1 -> output1/1
  Constant2/1 -> output2/1
  Constant3/1 -> output3/1
  Constant4/1 -> output4/1
  Constant5/1 -> output5/1
  Constant6/1 -> output6/1
  Constant7/1 -> output7/1
  Constant8/1 -> output8/1

== system six_plus_six_AcmsteeringV09_main_2lflm/Subsystem/VCU2/VCU1_GearCmd ==
  VCU1_GearCmd : Inport
  Constant{2..8} (7 alike) : Constant  Value=0  OutDataTypeStr=uint8
  VCU1_GearCmdRon : Rounding  Operator=round
  VCU1_GearCmd_1sat : Saturate  UpperLimit=24  LowerLimit=0
  VCU1_GearCmd_Convert : DataTypeConversion  OutDataTypeStr=uint8
  VCU1_GearCmd_Convert1 : DataTypeConversion  OutDataTypeStr=uint32
  VCU1_GearCmd_D : Product  Inputs=*/
  VCU1_GearCmd_F : Constant  OutDataTypeStr=single
  VCU1_GearCmd_L : simulink/Logic and Bit Operations/Bitwise Operator  logicop=AND  UseBitMask=on  BitMask=24  BitMaskRealWorld=Stored Integer
  VCU1_GearCmd_O : Constant  Value=0  OutDataTypeStr=single
  VCU1_GearCmd_S : ArithShift  BitShiftNumber=-3
  VCU1_GearCmd_sat : Saturate  UpperLimit=3  LowerLimit=0
  VCU1_GearCmd_st : Sum  Inputs=+-
  output1 : Outport
  output2 : Outport  Port=2
  output3 : Outport  Port=3
  output4 : Outport  Port=4
  output5 : Outport  Port=5
  output6 : Outport  Port=6
  output7 : Outport  Port=7
  output8 : Outport  Port=8
  wires:
  VCU1_GearCmd/1 -> VCU1_GearCmd_sat/1
  VCU1_GearCmd_sat/1 -> VCU1_GearCmd_st/1
  VCU1_GearCmd_O/1 -> VCU1_GearCmd_st/2
  VCU1_GearCmd_st/1 -> VCU1_GearCmd_D/1
  VCU1_GearCmd_F/1 -> VCU1_GearCmd_D/2
  VCU1_GearCmd_D/1 -> VCU1_GearCmdRon/1
  VCU1_GearCmdRon/1 -> VCU1_GearCmd_S/1
  VCU1_GearCmd_S/1 -> VCU1_GearCmd_1sat/1
  VCU1_GearCmd_1sat/1 -> VCU1_GearCmd_Convert1/1
  VCU1_GearCmd_Convert1/1 -> VCU1_GearCmd_L/1
  VCU1_GearCmd_L/1 -> VCU1_GearCmd_Convert/1
  VCU1_GearCmd_Convert/1 -> output1/1
  Constant2/1 -> output2/1
  Constant3/1 -> output3/1
  Constant4/1 -> output4/1
  Constant5/1 -> output5/1
  Constant6/1 -> output6/1
  Constant7/1 -> output7/1
  Constant8/1 -> output8/1

== system six_plus_six_AcmsteeringV09_main_2lflm/Subsystem/VCU2/VCU1_LifeCnt ==
  VCU1_LifeCnt : Inport
  Constant{1..7} (7 alike) : Constant  Value=0  OutDataTypeStr=uint8
  VCU1_LifeCntRon : Rounding  Operator=round
  VCU1_LifeCnt_1sat : Saturate  UpperLimit=255  LowerLimit=0
  VCU1_LifeCnt_Convert : DataTypeConversion  OutDataTypeStr=uint8
  VCU1_LifeCnt_Convert1 : DataTypeConversion  OutDataTypeStr=uint32
  VCU1_LifeCnt_D : Product  Inputs=*/
  VCU1_LifeCnt_F : Constant  OutDataTypeStr=single
  VCU1_LifeCnt_L : simulink/Logic and Bit Operations/Bitwise Operator  logicop=AND  UseBitMask=on  BitMask=255  BitMaskRealWorld=Stored Integer
  VCU1_LifeCnt_O : Constant  Value=0  OutDataTypeStr=single
  VCU1_LifeCnt_S : ArithShift
  VCU1_LifeCnt_sat : Saturate  UpperLimit=255  LowerLimit=0
  VCU1_LifeCnt_st : Sum  Inputs=+-
  output1 : Outport
  output2 : Outport  Port=2
  output3 : Outport  Port=3
  output4 : Outport  Port=4
  output5 : Outport  Port=5
  output6 : Outport  Port=6
  output7 : Outport  Port=7
  output8 : Outport  Port=8
  wires:
  VCU1_LifeCnt/1 -> VCU1_LifeCnt_sat/1
  VCU1_LifeCnt_sat/1 -> VCU1_LifeCnt_st/1
  VCU1_LifeCnt_O/1 -> VCU1_LifeCnt_st/2
  VCU1_LifeCnt_st/1 -> VCU1_LifeCnt_D/1
  VCU1_LifeCnt_F/1 -> VCU1_LifeCnt_D/2
  VCU1_LifeCnt_D/1 -> VCU1_LifeCntRon/1
  VCU1_LifeCntRon/1 -> VCU1_LifeCnt_S/1
  VCU1_LifeCnt_S/1 -> VCU1_LifeCnt_1sat/1
  VCU1_LifeCnt_1sat/1 -> VCU1_LifeCnt_Convert1/1
  VCU1_LifeCnt_Convert1/1 -> VCU1_LifeCnt_L/1
  VCU1_LifeCnt_L/1 -> VCU1_LifeCnt_Convert/1
  VCU1_LifeCnt_Convert/1 -> output8/1
  Constant1/1 -> output1/1
  Constant2/1 -> output2/1
  Constant3/1 -> output3/1
  Constant4/1 -> output4/1
  Constant5/1 -> output5/1
  Constant6/1 -> output6/1
  Constant7/1 -> output7/1

== system six_plus_six_AcmsteeringV09_main_2lflm/Subsystem/VCU2/VCU1_SpeedMax ==
  VCU1_SpeedMax : Inport
  Constant{1,4..8} (6 alike) : Constant  Value=0  OutDataTypeStr=uint8
  VCU1_SpeedMaxBitCov : DataTypeConversion  OutDataTypeStr=uint8
  VCU1_SpeedMaxCOV : DataTypeConversion  OutDataTypeStr=uint8
  VCU1_SpeedMaxRon : Rounding  Operator=round
  VCU1_SpeedMax_1sat : Saturate  UpperLimit=65535  LowerLimit=0
  VCU1_SpeedMax_And : simulink/Logic and Bit Operations/Bitwise Operator  logicop=AND  UseBitMask=off  NumInputPorts=2  BitMask=bin2dec('11011001')  BitMaskRealWorld=Stored Integer
  VCU1_SpeedMax_And_C : Constant  Value=255  OutDataTypeStr=uint32
  VCU1_SpeedMax_Convert : DataTypeConversion  OutDataTypeStr=uint32
  VCU1_SpeedMax_D : Product  Inputs=*/
  VCU1_SpeedMax_D1 : Product  Inputs=*/
  VCU1_SpeedMax_F : Constant  OutDataTypeStr=single
  VCU1_SpeedMax_L : simulink/Logic and Bit Operations/Bitwise Operator  logicop=AND  UseBitMask=on  BitMask=65535  BitMaskRealWorld=Stored Integer
  VCU1_SpeedMax_O : Constant  Value=0  OutDataTypeStr=single
  VCU1_SpeedMax_S : ArithShift
  VCU1_SpeedMax_sat : Saturate  UpperLimit=10000  LowerLimit=0
  VCU1_SpeedMax_st : Sum  Inputs=+-
  VCU1_SpeedMaxoutput2_C : Constant  Value=256
  output1 : Outport
  output2 : Outport  Port=2
  output3 : Outport  Port=3
  output4 : Outport  Port=4
  output5 : Outport  Port=5
  output6 : Outport  Port=6
  output7 : Outport  Port=7
  output8 : Outport  Port=8
  wires:
  VCU1_SpeedMax/1 -> VCU1_SpeedMax_sat/1
  VCU1_SpeedMax_sat/1 -> VCU1_SpeedMax_st/1
  VCU1_SpeedMax_O/1 -> VCU1_SpeedMax_st/2
  VCU1_SpeedMax_st/1 -> VCU1_SpeedMax_D/1
  VCU1_SpeedMax_F/1 -> VCU1_SpeedMax_D/2
  VCU1_SpeedMax_D/1 -> VCU1_SpeedMaxRon/1
  VCU1_SpeedMaxRon/1 -> VCU1_SpeedMax_S/1
  VCU1_SpeedMax_S/1 -> VCU1_SpeedMax_1sat/1
  VCU1_SpeedMax_1sat/1 -> VCU1_SpeedMax_Convert/1
  VCU1_SpeedMax_Convert/1 -> VCU1_SpeedMax_L/1
  VCU1_SpeedMax_L/1 -> VCU1_SpeedMax_D1/1, VCU1_SpeedMax_And/1
  VCU1_SpeedMaxoutput2_C/1 -> VCU1_SpeedMax_D1/2
  VCU1_SpeedMax_D1/1 -> VCU1_SpeedMaxCOV/1
  VCU1_SpeedMaxCOV/1 -> output2/1
  VCU1_SpeedMax_And_C/1 -> VCU1_SpeedMax_And/2
  VCU1_SpeedMax_And/1 -> VCU1_SpeedMaxBitCov/1
  VCU1_SpeedMaxBitCov/1 -> output3/1
  Constant1/1 -> output1/1
  Constant4/1 -> output4/1
  Constant5/1 -> output5/1
  Constant6/1 -> output6/1
  Constant7/1 -> output7/1
  Constant8/1 -> output8/1

== system six_plus_six_AcmsteeringV09_main_2lflm/Subsystem/VCU2/VCU1_TorqueRef ==
  VCU1_TorqueRef : Inport
  Constant{1..3,6..8} (6 alike) : Constant  Value=0  OutDataTypeStr=uint8
  VCU1_TorqueRefBitCov : DataTypeConversion  OutDataTypeStr=uint8
  VCU1_TorqueRefCOV : DataTypeConversion  OutDataTypeStr=uint8
  VCU1_TorqueRefRon : Rounding  Operator=round
  VCU1_TorqueRef_1sat : Saturate  UpperLimit=65535  LowerLimit=0
  VCU1_TorqueRef_And : simulink/Logic and Bit Operations/Bitwise Operator  logicop=AND  UseBitMask=off  NumInputPorts=2  BitMask=bin2dec('11011001')  BitMaskRealWorld=Stored Integer
  VCU1_TorqueRef_And_C : Constant  Value=255  OutDataTypeStr=uint32
  VCU1_TorqueRef_Convert : DataTypeConversion  OutDataTypeStr=uint32
  VCU1_TorqueRef_D : Product  Inputs=*/
  VCU1_TorqueRef_D1 : Product  Inputs=*/
  VCU1_TorqueRef_F : Constant  Value=0.1  OutDataTypeStr=single
  VCU1_TorqueRef_L : simulink/Logic and Bit Operations/Bitwise Operator  logicop=AND  UseBitMask=on  BitMask=65535  BitMaskRealWorld=Stored Integer
  VCU1_TorqueRef_O : Constant  Value=-1000  OutDataTypeStr=single
  VCU1_TorqueRef_S : ArithShift
  VCU1_TorqueRef_sat : Saturate  UpperLimit=1000  LowerLimit=-1000
  VCU1_TorqueRef_st : Sum  Inputs=+-
  VCU1_TorqueRefoutput4_C : Constant  Value=256
  output1 : Outport
  output2 : Outport  Port=2
  output3 : Outport  Port=3
  output4 : Outport  Port=4
  output5 : Outport  Port=5
  output6 : Outport  Port=6
  output7 : Outport  Port=7
  output8 : Outport  Port=8
  wires:
  VCU1_TorqueRef/1 -> VCU1_TorqueRef_sat/1
  VCU1_TorqueRef_sat/1 -> VCU1_TorqueRef_st/1
  VCU1_TorqueRef_O/1 -> VCU1_TorqueRef_st/2
  VCU1_TorqueRef_st/1 -> VCU1_TorqueRef_D/1
  VCU1_TorqueRef_F/1 -> VCU1_TorqueRef_D/2
  VCU1_TorqueRef_D/1 -> VCU1_TorqueRefRon/1
  VCU1_TorqueRefRon/1 -> VCU1_TorqueRef_S/1
  VCU1_TorqueRef_S/1 -> VCU1_TorqueRef_1sat/1
  VCU1_TorqueRef_1sat/1 -> VCU1_TorqueRef_Convert/1
  VCU1_TorqueRef_Convert/1 -> VCU1_TorqueRef_L/1
  VCU1_TorqueRef_L/1 -> VCU1_TorqueRef_D1/1, VCU1_TorqueRef_And/1
  VCU1_TorqueRefoutput4_C/1 -> VCU1_TorqueRef_D1/2
  VCU1_TorqueRef_D1/1 -> VCU1_TorqueRefCOV/1
  VCU1_TorqueRefCOV/1 -> output4/1
  VCU1_TorqueRef_And_C/1 -> VCU1_TorqueRef_And/2
  VCU1_TorqueRef_And/1 -> VCU1_TorqueRefBitCov/1
  VCU1_TorqueRefBitCov/1 -> output5/1
  Constant1/1 -> output1/1
  Constant2/1 -> output2/1
  Constant3/1 -> output3/1
  Constant6/1 -> output6/1
  Constant7/1 -> output7/1
  Constant8/1 -> output8/1

== system six_plus_six_AcmsteeringV09_main_2lflm/Subsystem/VCU3/VCU1_CtrlModel ==
  VCU1_CtrlModel : Inport
  Constant{2..8} (7 alike) : Constant  Value=0  OutDataTypeStr=uint8
  VCU1_CtrlModelRon : Rounding  Operator=round
  VCU1_CtrlModel_1sat : Saturate  UpperLimit=4  LowerLimit=0
  VCU1_CtrlModel_Convert : DataTypeConversion  OutDataTypeStr=uint8
  VCU1_CtrlModel_Convert1 : DataTypeConversion  OutDataTypeStr=uint32
  VCU1_CtrlModel_D : Product  Inputs=*/
  VCU1_CtrlModel_F : Constant  OutDataTypeStr=single
  VCU1_CtrlModel_L : simulink/Logic and Bit Operations/Bitwise Operator  logicop=AND  UseBitMask=on  BitMask=4  BitMaskRealWorld=Stored Integer
  VCU1_CtrlModel_O : Constant  Value=0  OutDataTypeStr=single
  VCU1_CtrlModel_S : ArithShift  BitShiftNumber=-2
  VCU1_CtrlModel_sat : Saturate  UpperLimit=1  LowerLimit=0
  VCU1_CtrlModel_st : Sum  Inputs=+-
  output1 : Outport
  output2 : Outport  Port=2
  output3 : Outport  Port=3
  output4 : Outport  Port=4
  output5 : Outport  Port=5
  output6 : Outport  Port=6
  output7 : Outport  Port=7
  output8 : Outport  Port=8
  wires:
  VCU1_CtrlModel/1 -> VCU1_CtrlModel_sat/1
  VCU1_CtrlModel_sat/1 -> VCU1_CtrlModel_st/1
  VCU1_CtrlModel_O/1 -> VCU1_CtrlModel_st/2
  VCU1_CtrlModel_st/1 -> VCU1_CtrlModel_D/1
  VCU1_CtrlModel_F/1 -> VCU1_CtrlModel_D/2
  VCU1_CtrlModel_D/1 -> VCU1_CtrlModelRon/1
  VCU1_CtrlModelRon/1 -> VCU1_CtrlModel_S/1
  VCU1_CtrlModel_S/1 -> VCU1_CtrlModel_1sat/1
  VCU1_CtrlModel_1sat/1 -> VCU1_CtrlModel_Convert1/1
  VCU1_CtrlModel_Convert1/1 -> VCU1_CtrlModel_L/1
  VCU1_CtrlModel_L/1 -> VCU1_CtrlModel_Convert/1
  VCU1_CtrlModel_Convert/1 -> output1/1
  Constant2/1 -> output2/1
  Constant3/1 -> output3/1
  Constant4/1 -> output4/1
  Constant5/1 -> output5/1
  Constant6/1 -> output6/1
  Constant7/1 -> output7/1
  Constant8/1 -> output8/1

== system six_plus_six_AcmsteeringV09_main_2lflm/Subsystem/VCU3/VCU1_EnableReq ==
  VCU1_EnableReq : Inport
  Constant{2..8} (7 alike) : Constant  Value=0  OutDataTypeStr=uint8
  VCU1_EnableReqRon : Rounding  Operator=round
  VCU1_EnableReq_1sat : Saturate  UpperLimit=3  LowerLimit=0
  VCU1_EnableReq_Convert : DataTypeConversion  OutDataTypeStr=uint8
  VCU1_EnableReq_Convert1 : DataTypeConversion  OutDataTypeStr=uint32
  VCU1_EnableReq_D : Product  Inputs=*/
  VCU1_EnableReq_F : Constant  OutDataTypeStr=single
  VCU1_EnableReq_L : simulink/Logic and Bit Operations/Bitwise Operator  logicop=AND  UseBitMask=on  BitMask=3  BitMaskRealWorld=Stored Integer
  VCU1_EnableReq_O : Constant  Value=0  OutDataTypeStr=single
  VCU1_EnableReq_S : ArithShift
  VCU1_EnableReq_sat : Saturate  UpperLimit=3  LowerLimit=0
  VCU1_EnableReq_st : Sum  Inputs=+-
  output1 : Outport
  output2 : Outport  Port=2
  output3 : Outport  Port=3
  output4 : Outport  Port=4
  output5 : Outport  Port=5
  output6 : Outport  Port=6
  output7 : Outport  Port=7
  output8 : Outport  Port=8
  wires:
  VCU1_EnableReq/1 -> VCU1_EnableReq_sat/1
  VCU1_EnableReq_sat/1 -> VCU1_EnableReq_st/1
  VCU1_EnableReq_O/1 -> VCU1_EnableReq_st/2
  VCU1_EnableReq_st/1 -> VCU1_EnableReq_D/1
  VCU1_EnableReq_F/1 -> VCU1_EnableReq_D/2
  VCU1_EnableReq_D/1 -> VCU1_EnableReqRon/1
  VCU1_EnableReqRon/1 -> VCU1_EnableReq_S/1
  VCU1_EnableReq_S/1 -> VCU1_EnableReq_1sat/1
  VCU1_EnableReq_1sat/1 -> VCU1_EnableReq_Convert1/1
  VCU1_EnableReq_Convert1/1 -> VCU1_EnableReq_L/1
  VCU1_EnableReq_L/1 -> VCU1_EnableReq_Convert/1
  VCU1_EnableReq_Convert/1 -> output1/1
  Constant2/1 -> output2/1
  Constant3/1 -> output3/1
  Constant4/1 -> output4/1
  Constant5/1 -> output5/1
  Constant6/1 -> output6/1
  Constant7/1 -> output7/1
  Constant8/1 -> output8/1

== system six_plus_six_AcmsteeringV09_main_2lflm/Subsystem/VCU3/VCU1_GearCmd ==
  VCU1_GearCmd : Inport
  Constant{2..8} (7 alike) : Constant  Value=0  OutDataTypeStr=uint8
  VCU1_GearCmdRon : Rounding  Operator=round
  VCU1_GearCmd_1sat : Saturate  UpperLimit=24  LowerLimit=0
  VCU1_GearCmd_Convert : DataTypeConversion  OutDataTypeStr=uint8
  VCU1_GearCmd_Convert1 : DataTypeConversion  OutDataTypeStr=uint32
  VCU1_GearCmd_D : Product  Inputs=*/
  VCU1_GearCmd_F : Constant  OutDataTypeStr=single
  VCU1_GearCmd_L : simulink/Logic and Bit Operations/Bitwise Operator  logicop=AND  UseBitMask=on  BitMask=24  BitMaskRealWorld=Stored Integer
  VCU1_GearCmd_O : Constant  Value=0  OutDataTypeStr=single
  VCU1_GearCmd_S : ArithShift  BitShiftNumber=-3
  VCU1_GearCmd_sat : Saturate  UpperLimit=3  LowerLimit=0
  VCU1_GearCmd_st : Sum  Inputs=+-
  output1 : Outport
  output2 : Outport  Port=2
  output3 : Outport  Port=3
  output4 : Outport  Port=4
  output5 : Outport  Port=5
  output6 : Outport  Port=6
  output7 : Outport  Port=7
  output8 : Outport  Port=8
  wires:
  VCU1_GearCmd/1 -> VCU1_GearCmd_sat/1
  VCU1_GearCmd_sat/1 -> VCU1_GearCmd_st/1
  VCU1_GearCmd_O/1 -> VCU1_GearCmd_st/2
  VCU1_GearCmd_st/1 -> VCU1_GearCmd_D/1
  VCU1_GearCmd_F/1 -> VCU1_GearCmd_D/2
  VCU1_GearCmd_D/1 -> VCU1_GearCmdRon/1
  VCU1_GearCmdRon/1 -> VCU1_GearCmd_S/1
  VCU1_GearCmd_S/1 -> VCU1_GearCmd_1sat/1
  VCU1_GearCmd_1sat/1 -> VCU1_GearCmd_Convert1/1
  VCU1_GearCmd_Convert1/1 -> VCU1_GearCmd_L/1
  VCU1_GearCmd_L/1 -> VCU1_GearCmd_Convert/1
  VCU1_GearCmd_Convert/1 -> output1/1
  Constant2/1 -> output2/1
  Constant3/1 -> output3/1
  Constant4/1 -> output4/1
  Constant5/1 -> output5/1
  Constant6/1 -> output6/1
  Constant7/1 -> output7/1
  Constant8/1 -> output8/1

== system six_plus_six_AcmsteeringV09_main_2lflm/Subsystem/VCU3/VCU1_LifeCnt ==
  VCU1_LifeCnt : Inport
  Constant{1..7} (7 alike) : Constant  Value=0  OutDataTypeStr=uint8
  VCU1_LifeCntRon : Rounding  Operator=round
  VCU1_LifeCnt_1sat : Saturate  UpperLimit=255  LowerLimit=0
  VCU1_LifeCnt_Convert : DataTypeConversion  OutDataTypeStr=uint8
  VCU1_LifeCnt_Convert1 : DataTypeConversion  OutDataTypeStr=uint32
  VCU1_LifeCnt_D : Product  Inputs=*/
  VCU1_LifeCnt_F : Constant  OutDataTypeStr=single
  VCU1_LifeCnt_L : simulink/Logic and Bit Operations/Bitwise Operator  logicop=AND  UseBitMask=on  BitMask=255  BitMaskRealWorld=Stored Integer
  VCU1_LifeCnt_O : Constant  Value=0  OutDataTypeStr=single
  VCU1_LifeCnt_S : ArithShift
  VCU1_LifeCnt_sat : Saturate  UpperLimit=255  LowerLimit=0
  VCU1_LifeCnt_st : Sum  Inputs=+-
  output1 : Outport
  output2 : Outport  Port=2
  output3 : Outport  Port=3
  output4 : Outport  Port=4
  output5 : Outport  Port=5
  output6 : Outport  Port=6
  output7 : Outport  Port=7
  output8 : Outport  Port=8
  wires:
  VCU1_LifeCnt/1 -> VCU1_LifeCnt_sat/1
  VCU1_LifeCnt_sat/1 -> VCU1_LifeCnt_st/1
  VCU1_LifeCnt_O/1 -> VCU1_LifeCnt_st/2
  VCU1_LifeCnt_st/1 -> VCU1_LifeCnt_D/1
  VCU1_LifeCnt_F/1 -> VCU1_LifeCnt_D/2
  VCU1_LifeCnt_D/1 -> VCU1_LifeCntRon/1
  VCU1_LifeCntRon/1 -> VCU1_LifeCnt_S/1
  VCU1_LifeCnt_S/1 -> VCU1_LifeCnt_1sat/1
  VCU1_LifeCnt_1sat/1 -> VCU1_LifeCnt_Convert1/1
  VCU1_LifeCnt_Convert1/1 -> VCU1_LifeCnt_L/1
  VCU1_LifeCnt_L/1 -> VCU1_LifeCnt_Convert/1
  VCU1_LifeCnt_Convert/1 -> output8/1
  Constant1/1 -> output1/1
  Constant2/1 -> output2/1
  Constant3/1 -> output3/1
  Constant4/1 -> output4/1
  Constant5/1 -> output5/1
  Constant6/1 -> output6/1
  Constant7/1 -> output7/1
